simulink model "pll02"  (Simulink 8.1)
settings: Solver=ode45  StartTime=0.0  StopTime=10  MaxStep=0.0001  RelTol=1e-3
undefined symbols (not defined in the file or in its folder): fdesignblkfcn, gcbh
libraries: commsynccomp2 x1, commnoisgen2 x1, simulink x1
settings Model: Creator=my88899  LastModifiedBy=my88899
settings DataIOCC: SignalLoggingSaveFormat=Dataset
settings OptimizationCC: ExpressionDepthLimit=128
settings DebuggingCC: FcnCallInpInsideContextMsg=EnableAllAsError
settings GRTTargetCC: CombineOutputUpdateFcns=on  GRTInterface=off

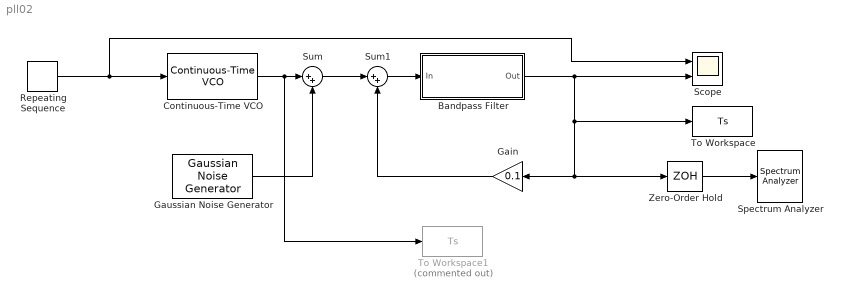
== system pll02 ==
  Bandpass Filter : Subsystem  DialogController=fdesignblkfcn  DialogControllerArgs=DataTag1  InitFcn=fdesignblkfcn(gcbh, {'InitFcn'});  mask(Bandpass Filter){}
      mask help: Design a bandpass filter
      settings: CopyFcn=fdesignblkfcn(gcbh, {'CopyFcn'});
      mask Help: helpview(mapfilelocation('dsp'), 'dspbandpassfilter');
      mask Display: disp('Bandpass');
  Continuous-Time VCO : commsynccomp2/Continuous-Time VCO  Ac=5  Fc=100  Kc=100  Ph=0
  Gain : Gain  Gain=0.1
  Gaussian Noise Generator : commnoisgen2/Gaussian Noise Generator  m=0  d=1  s=2333  Ts=0.1  frameBased=off  sampPerFrame=1  orient=off  outDataType=double
  Repeating Sequence : simulink/Sources/Repeating Sequence  rep_seq_t=[0 1]  rep_seq_y=[0 5]
  Scope : Scope  NumInputPorts=2
      settings: TimeRange=0.1038961038961048  YMin=5.645~-5  YMax=5.7~5  MaxDataPoints=100000
  Spectrum Analyzer : SpectrumAnalyzer
      settings: CopyFcn=scopeextensions.ScopeBlock.callback(gcbh, 'onBlockCopy', gcbh);  DeleteFcn=scopeextensions.ScopeBlock.callback(gcbh, 'onBlockDelete');  PreSaveFcn=scopeextensions.ScopeBlock.callback(gcbh, 'onModelSave');  NameChangeFcn=scopeextensions.ScopeBlock.callback(gcbh, 'onBlockRename');  CloseFcn=scopeextensions.ScopeBlock.callback(gcbh, 'onBlockClose');  PreDeleteFcn=scopeextensions.ScopeBlock.callback(gcbh, 'onBlockPreDelete');
  Sum : Sum  Inputs=|++
  Sum1 : Sum  Inputs=|++
  To Workspace : ToWorkspace  VariableName=Ts  SampleTime=-1  SaveFormat=Timeseries
  To Workspace1 : ToWorkspace  Commented=on  VariableName=Ts  SampleTime=-1  SaveFormat=Timeseries
  Zero-Order Hold : ZeroOrderHold  SampleTime=0.01
  wires:
  Repeating Sequence/1 -> Scope/1, Continuous-Time VCO/1
  Zero-Order Hold/1 -> Spectrum Analyzer/1
  Gain/1 -> Sum1/2
  Continuous-Time VCO/1 -> To Workspace1/1, Sum/1
  Sum/1 -> Sum1/1
  Sum1/1 -> Bandpass Filter/1(In)
  Gaussian Noise Generator/1 -> Sum/2
  Bandpass Filter/1(Out) -> Scope/2, To Workspace/1, Zero-Order Hold/1, Gain/1

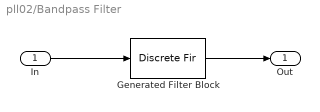
== system pll02/Bandpass Filter ==
  In : Inport
  Generated Filter Block : DiscreteFir  Tag=BlockMethodSubSystem  Coefficients=[-0.00075942703500712764 0.0037090301386008924 -0.0033106226162894041 -0.021329161407229749 -0.0076722244057639555 0.0096874334248229881 -0.0030281918306349328 0.0051220881712012879 0.012613452200942723 -0.0010552570293253314 0.014916575663563417 0.013836009896681154 0.00073417238967297873 0.023080028394343859 0.0075804666812208932 -0.00023681597941664287 0.023619662812307193 -0.01059274166774048 -0.0049336642388191597 0.011591199545326027 -0.04074287877026872 -0.010621441117850784 -0.015153507227397927 -0.077379310026114215 -0.0090520904546812671 -0.058123414524053618 -0.11081592621032275 0.022180131177871192 -0.14329612169488204 -0.13080390605868614 0.50073126282405578 0.50073126282405578 -0.13080390605868614 -0.14329612169488204 0.022180131177871192 -0.11081592621032275 -0.058123414524053618 -0.0090520904546812671 -0.077379310026114215 -0.015153507227397927 -0.010621441117850784 -0.04074287877026872 0.011591199545326027 -0.0049336642388191597 -0.01059274166774048 0.023619662812307193 -0.00023681597941664287 0.0075804666812208932 0.023080028394343859 0.00073417238967297873 0.013836009896681154 0.014916575663563417 -0.0010552570293253314 0.012613452200942723 0.0051220881712012879 -0.0030281918306349328 0.0096874334248229881 -0.0076722244057639555 -0.021329161407229749 -0.0033106226162894041 0.0037090301386008924 -0.00075942703500712764]  InputProcessing=Columns as channels (frame based)
  Out : Outport
  wires:
  In/1 -> Generated Filter Block/1
  Generated Filter Block/1 -> Out/1
